simulink model "A1_9_openloop_ramp_input"  (Simulink 7.4)
settings: Solver=FixedStepDiscrete  StartTime=0.0  StopTime=10.0  RelTol=1e-3
libraries: DCmotor_library x1, simulink x1
settings Model: Creator=Patrick  LastModifiedBy=ma
settings OptimizationCC: ExpressionDepthLimit=128
settings DebuggingCC: FcnCallInpInsideContextMsg=Enable All  StrictBusMsg=ErrorLevel1
settings CodeAppCC: CustomSymbolStrType=$N$R$M_T
settings GRTTargetCC: CombineOutputUpdateFcns=on

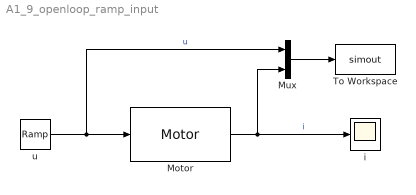
== system A1_9_openloop_ramp_input ==
  Motor : DCmotor_library/Motor  motoridinput=1  name_signal=Current  ts=10
  Mux : Mux  Inputs=2
  To Workspace : ToWorkspace  VariableName=simout  SampleTime=-1  SaveFormat=Structure With Time
  i : Scope
      settings: YMin=-8.67362e-19  YMax=0.035
  u : simulink/Sources/Ramp  slope=0.5  start=0  X0=0
  wires:
  Motor/1 -> Mux/2, i/1  "i"
  u/1 -> Mux/1, Motor/1  "u"
  Mux/1 -> To Workspace/1
